simulink model "FormaDir2"  (R2020b)
settings: Solver=VariableStepAuto  StartTime=0.0  StopTime=40.0  RelTol=1e-3
libraries: dspsnks4 x1, dspvision x1
settings Model: Creator=Nic  LastModifiedBy=Nic

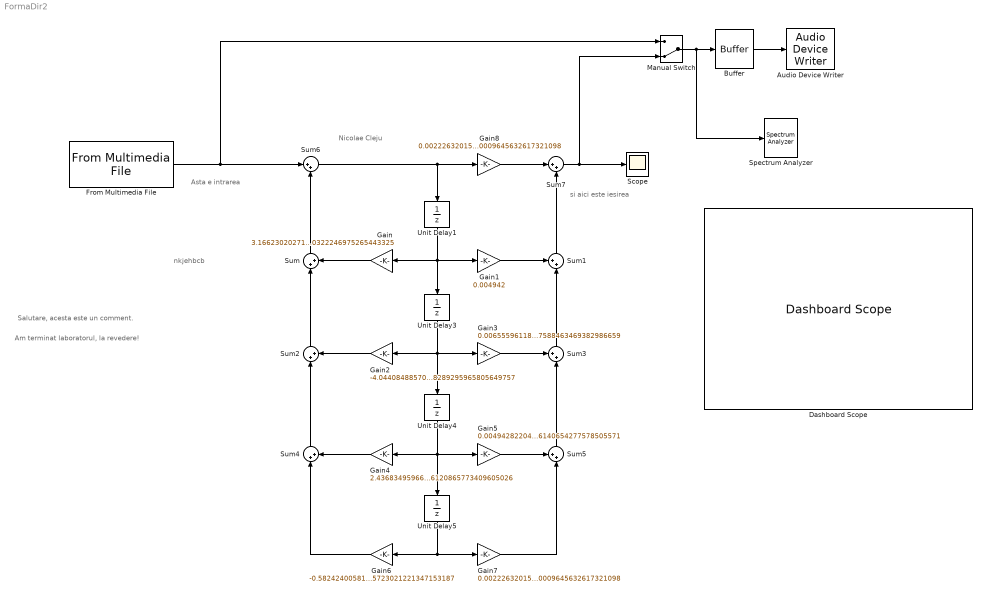
== system FormaDir2 ==
  note: Am terminat laboratorul, la revedere!
  note: Salutare, acesta este un comment.
  note: nkjehbcb
  note: si aici este iesirea
  note: Asta e intrarea
  note: Nicolae Cleju
  Audio Device Writer : dspsnks4/Audio Device Writer  Driver=DirectSound  Device=Default  InheritSampleRate=on  SampleRate=44100  BitDepth=16-bit integer  BufferSize=4096  NumBuffers=10  DefaultOutputChannelMapping=on  OutputChannelMapping=1:2  OutputNumUnderrunSamples=off  DriverIdx=1  DeviceWarnFlag=''
  Buffer : Buffer  N=1024  OutputFrames=off
  Dashboard Scope : DashboardScope
  From Multimedia File : dspvision/From Multimedia File  inputFilename=D:\2020_2021\PSS\Work\L04_5406\Labs_Sample.wav  readRange=[1 Inf]  loop=on  numPlays=inf  outputStreams=Audio only  videoDataType=single  audioDataType=double  inheritSampleTime=on  userDefinedSampleTime=1/30  noAudioOutput=off  isIntensityVideo=off  fourcc=RGB  colorVideoFormat=One multidimensional signal  outputEOF=off  dataOrg=Column-major  audioFrameSize=1  computeAudioFrameSize=off  outSamplingMode=Sample based
  Gain : Gain  Gain=3.166230202716211916680322246975265443325
  Gain1 : Gain  Gain=0.004942
  Gain2 : Gain  Gain=-4.044084885701303200278289295965805649757
  Gain3 : Gain  Gain=0.006555961183574801967588463469382986659
  Gain4 : Gain  Gain=2.436834959662190769336120865773409605026
  Gain5 : Gain  Gain=0.0049428220453378406140654277578505571
  Gain6 : Gain  Gain=-0.582424005814285994375723021221347153187
  Gain7 : Gain  Gain=0.002226320156310144030009645632617321098
  Gain8 : Gain  Gain=0.002226320156310144030009645632617321098
  Manual Switch : ManualSwitch  CurrentSetting=0
  Scope : Scope
  Spectrum Analyzer : SpectrumAnalyzer
  Sum{,2,4,6..7} (5 alike) : Sum  Inputs=|++
  Sum1 : Sum  Inputs=++|
  Sum3 : Sum  Inputs=++|
  Sum5 : Sum  Inputs=++|
  Unit Delay{1,3..5} (4 alike) : UnitDelay  SampleTime=-1  HasFrameUpgradeWarning=on
  wires:
  Unit Delay1/1 -> Unit Delay3/1, Gain1/1, Gain/1
  Gain/1 -> Sum/2
  Gain1/1 -> Sum1/1
  Unit Delay3/1 -> Unit Delay4/1, Gain3/1, Gain2/1
  Gain2/1 -> Sum2/2
  Gain3/1 -> Sum3/1
  Unit Delay4/1 -> Unit Delay5/1, Gain5/1, Gain4/1
  Gain4/1 -> Sum4/2
  Gain5/1 -> Sum5/1
  Unit Delay5/1 -> Gain7/1, Gain6/1
  Gain6/1 -> Sum4/1
  Gain7/1 -> Sum5/2
  Sum4/1 -> Sum2/1
  Sum5/1 -> Sum3/2
  Sum2/1 -> Sum/1
  Sum3/1 -> Sum1/2
  Sum1/1 -> Sum7/2
  Sum/1 -> Sum6/2
  Sum6/1 -> Unit Delay1/1, Gain8/1
  From Multimedia File/1 -> Manual Switch/1, Sum6/1
  Sum7/1 -> Manual Switch/2, Scope/1
  Gain8/1 -> Sum7/1
  Buffer/1 -> Audio Device Writer/1
  Manual Switch/1 -> Spectrum Analyzer/1, Buffer/1
